simulink model "Receiver"  (Simulink 7.7)
settings: Solver=ode45  StartTime=0.0  StopTime=10  RelTol=1e-3
PreLoadFcn:
  | EbNo = 16; Errors = 188; Bits = 1e8; M = 256; N = 64; Ts = (1/22050); constellation; InnerInterleaverBitTable
undefined symbols (not defined in the file or in its folder): rsgenpoly
libraries: commblkintrlv2 x3, commblkcod2 x1, dspsnks4 x1, commutil2 x1, commcnvintrlv2 x1, dspsigops x1, commcnvcod2 x1, dspxfrm3 x1, commdigbbndam3 x1, commsdrhw_v2 x1
settings Model: Creator=katsikas  LastModifiedBy=katsikas
settings SimEventsCC: propDiagAttribOutput=1  propDiagFcnCallOutput=1  propDiagStatOutput=0

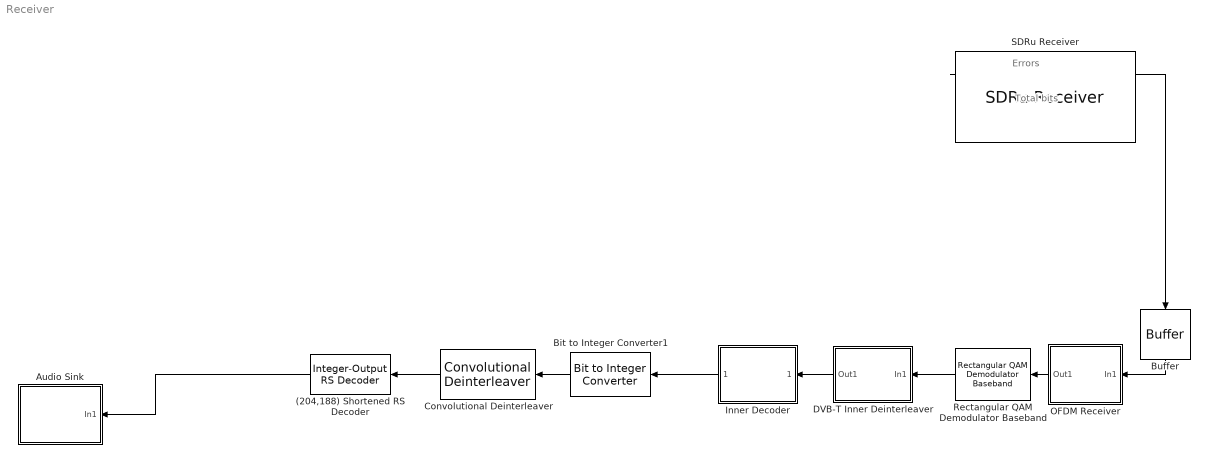
== system Receiver ==
  note: Total bits
  note: Errors
  (204,188) Shortened RS Decoder : commblkcod2/Integer-Output RS Decoder  n=204  k=188  specPrimPoly=off  prPoly=[1 0 1 1]  specGenPoly=off  genPoly=rsgenpoly(7,3)  specPuncture=off  punctVec=[ones(2,1); zeros(2,1)]  specErasurePort=off  showNumErr=off
  Audio Sink : Subsystem
  Bit to Integer Converter1 : commutil2/Bit to Integer Converter  nbits=log2(M)  bitOrder=MSB first  signedOutputValues=Unsigned  outDtype=uint8  outDtypeSigned=Inherit via internal rule
  Buffer : Buffer  N=2048  TreatMby1Signals=One channel
  Convolutional Deinterleaver : commcnvintrlv2/Convolutional Deinterleaver  SystemSampleTime=-1  N=12  B=17  ic=0
  DVB-T Inner Deinterleaver : Subsystem  mask(DVB-T Inner Deinterleaver){}
      mask init:
      | fullILVec = [(1:126) ...
      |  (rem([0:125]+63,126) +1 + 126     ) ...
      |  (rem([0:125]+105,126)+1 + (2*126) ) ...
      |  (rem([0:125]+42,126) +1 + (3*126) ) ...
      |  (rem([0:125]+21,126) +1 + (4*126) ) ...
      |  (rem([0:125]+84,126) +1 + (5*126) )];
      mask Display: disp('DVB-T\nInner\nDeinterleaver')
  Inner Decoder : Subsystem
      mask Display: disp('Viterbi\nDecoder')
  OFDM Receiver : Subsystem
  Rectangular QAM Demodulator Baseband : commdigbbndam3/Rectangular QAM Demodulator Baseband  M=N  PowType=Average Power  MinDist=2  AvgPow=1  PeakPow=1  Ph=0  Dec=User-defined  Mapping=map_constellation  OutType=Bit  DecType=Hard decision  VarSource=Dialog  Variance=1  outDtype1=boolean  outDtype2=Inherit via internal rule  derotateFactorWordLen=16  denormFactorWordLen=16  prodOutWordLen=32  prodOutRoundingMode=Floor  prodOutOverflowMode=Wrap  sumWordLen=32
  SDRu Receiver : commsdrhw_v2/SDRu Receiver  SystemSampleTime=-1  rxtx=rx  USRP2_IP='192.168.10.2'  centerFrequency=794e6  centerFrequencySrc=Dialog  loOffset=0  loOffsetSrc=Dialog  gain=20  gainSrc=Dialog  decimInterp=512  decimInterpSrc=Dialog  USRP2_IP_NUM=[49 57 50 46 49 54 56 46 49 48 46 50]  frameLength=2048*10000  outputDatatype=double  overrunUnderrunPort=off  sampleTime=1  HOST_DATA_PORT=0  HOST_CONTROL_PORT=0  USRP2_DATA_PORT=0  USRP2_CONTROL_PORT=0
  wires:
  (204,188) Shortened RS Decoder/1 -> Audio Sink/1(In1)
  Convolutional Deinterleaver/1 -> (204,188) Shortened RS Decoder/1
  Rectangular QAM Demodulator Baseband/1 -> DVB-T Inner Deinterleaver/1(In1)
  Bit to Integer Converter1/1 -> Convolutional Deinterleaver/1
  Inner Decoder/1(Decoded symbols) -> Bit to Integer Converter1/1
  DVB-T Inner Deinterleaver/1(Out1) -> Inner Decoder/1(Received bits)
  OFDM Receiver/1(Out1) -> Rectangular QAM Demodulator Baseband/1
  SDRu Receiver/1 -> Buffer/1
  Buffer/1 -> OFDM Receiver/1(In1)

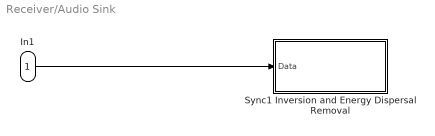
== system Receiver/Audio Sink ==
  In1 : Inport
  Sync1 Inversion and Energy Dispersal Removal : Subsystem
  wires:
  In1/1 -> Sync1 Inversion and Energy Dispersal Removal/1(Data)

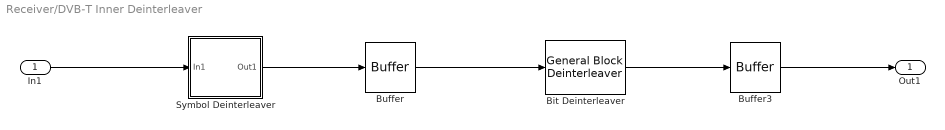
== system Receiver/DVB-T Inner Deinterleaver ==
  In1 : Inport
  Bit Deinterleaver : commblkintrlv2/General Block Deinterleaver  elements=BitInterleaverTable
  Buffer : Buffer  N=756  TreatMby1Signals=One channel
  Buffer3 : Buffer  N=2176  TreatMby1Signals=One channel
  Symbol Deinterleaver : Subsystem
      mask Display:
      | port_label('input', 1, '')
      | port_label('output', 1, '')
      | disp('Symbol\nDeinterleaver')
  Out1 : Outport
  wires:
  In1/1 -> Symbol Deinterleaver/1(In1)
  Buffer3/1 -> Out1/1
  Buffer/1 -> Bit Deinterleaver/1
  Bit Deinterleaver/1 -> Buffer3/1
  Symbol Deinterleaver/1(Out1) -> Buffer/1

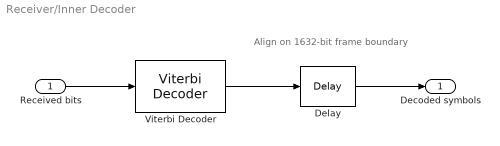
== system Receiver/Inner Decoder ==
  note: Align on 1632-bit
      | frame boundary
  Received bits : Inport
  Delay : dspsigops/Delay  InputProcessing=Columns as channels (frame based)  dly_unit=Samples  delay=584+69  ic_detail=off  dif_ic_for_ch=off  dif_ic_for_dly=off  ic=0  reset_popup=None
  Viterbi Decoder : commcnvcod2/Viterbi Decoder  trellis=poly2trellis(7, [171 133])  isPunctured=on  punctureVector=[1 1 0 1 1 0]'  erasures=off  dectype=Hard decision  runSigValErrCheck=off  nsdecb=4  smWordLength=16  tbdepth=136  opmode=Continuous  reset=off  outDataType=boolean
  Decoded symbols : Outport
  wires:
  Viterbi Decoder/1 -> Delay/1
  Received bits/1 -> Viterbi Decoder/1
  Delay/1 -> Decoded symbols/1

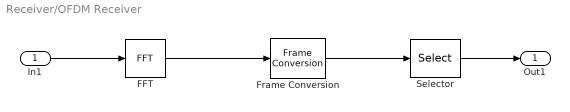
== system Receiver/OFDM Receiver ==
  In1 : Inport
  FFT : dspxfrm3/FFT  CompMethod=Table lookup  TableOpt=NEW  TableOptActive=Speed  BitRevOrder=off  InheritFFTLength=on  FFTLength=64  RowConvenienceOn=on  SkipNorm=off  firstCoeffDataTypeStr=Inherit: Same word length as input  firstCoeffLastDataTypeStr=Inherit: Same word length as input  outputMin=[]  outputMax=[]  roundingMode=Floor  overflowMode=off
  Frame Conversion : FrameConversion
  Selector : Selector  NumberOfDimensions=2  InputPortWidth=3  IndexOptions=Index vector (dialog),Select all  Indices=[1:756 1293:2048],1  OutputSizes=1,1
  Out1 : Outport
  wires:
  FFT/1 -> Frame Conversion/1
  Frame Conversion/1 -> Selector/1
  In1/1 -> FFT/1
  Selector/1 -> Out1/1

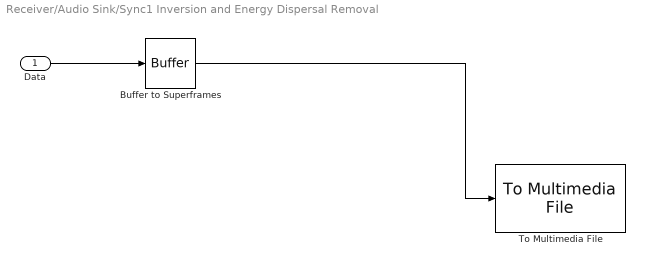
== system Receiver/Audio Sink/Sync1 Inversion and Energy Dispersal Removal ==
  Data : Inport
  Buffer to Superframes : Buffer  N=1504  TreatMby1Signals=One channel
  To Multimedia File : dspsnks4/To Multimedia File  outputFilename=output.avi  streamSelection=Video only  videoCompressor=None (uncompressed)  audioCompressor=None (uncompressed)  imagePorts=One multidimensional signal  fileType=AVI  audioDatatype=Determine from input data type  fourcc=RGB
  wires:
  Data/1 -> Buffer to Superframes/1
  Buffer to Superframes/1 -> To Multimedia File/1

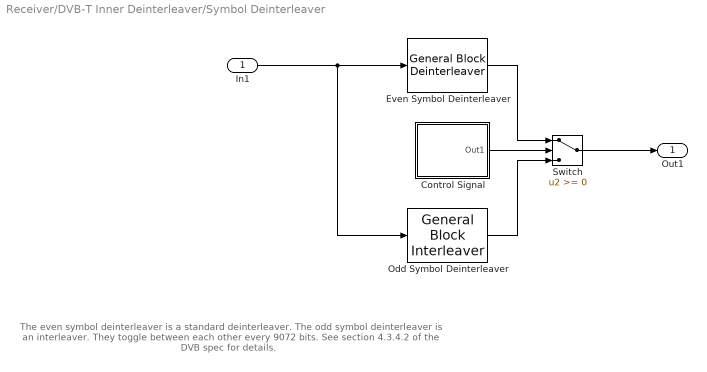
== system Receiver/DVB-T Inner Deinterleaver/Symbol Deinterleaver ==
  note: The even symbol deinterleaver is a standard deinterleaver.  The odd symbol deinterleaver is an interleaver.  They toggle
      | between each other every 9072 bits.  See section 4.3.4.2 of the DVB spec for details.
  In1 : Inport
  Control Signal : Subsystem
      mask Display:
      | port_label('output', 1, 'ctrl')
      | disp('Control\nSignal')
  Even Symbol Deinterleaver : commblkintrlv2/General Block Deinterleaver  elements=dvb_sym_int_table
  Odd Symbol Deinterleaver : commblkintrlv2/General Block Interleaver  elements=dvb_sym_int_table
  Switch : Switch
  Out1 : Outport
  wires:
  In1/1 -> Odd Symbol Deinterleaver/1, Even Symbol Deinterleaver/1
  Switch/1 -> Out1/1
  Control Signal/1(Out1) -> Switch/2
  Even Symbol Deinterleaver/1 -> Switch/1
  Odd Symbol Deinterleaver/1 -> Switch/3

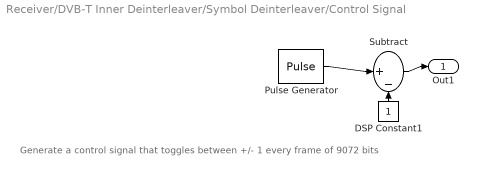
== system Receiver/DVB-T Inner Deinterleaver/Symbol Deinterleaver/Control Signal ==
  note: Generate a control signal that toggles between +/- 1 every frame of 9072 bits
  DSP Constant1 : Constant  VectorParams1D=off
  Pulse Generator : DiscretePulseGenerator  Amplitude=2  SampleTime=-1
  Subtract : Sum  Inputs=|+-
  Out1 : Outport
  wires:
  Subtract/1 -> Out1/1
  DSP Constant1/1 -> Subtract/2
  Pulse Generator/1 -> Subtract/1
